simulink model "MMC_detector"  (R2022b)
settings: Solver=VariableStepAuto  StartTime=0.0  StopTime=0.6  RelTol=1e-3
undefined symbols (not defined in the file or in its folder): Atk1, Atk2, Atk3, DiscIntNeverNeededParam, plecs, Tatk1, Tatk2, Ti, Ts, Tstop
libraries: simulink x6
settings Model: Creator=Asus  LastModifiedBy=ben19
settings DebuggingCC: UnconnectedInputMsg=warning  UnconnectedOutputMsg=warning  UnconnectedLineMsg=warning
settings ModelReferenceCC: EnableRefExpFcnMdlSchedulingChecks=on
settings RTWCC: DLArmComputeVersion=19.05

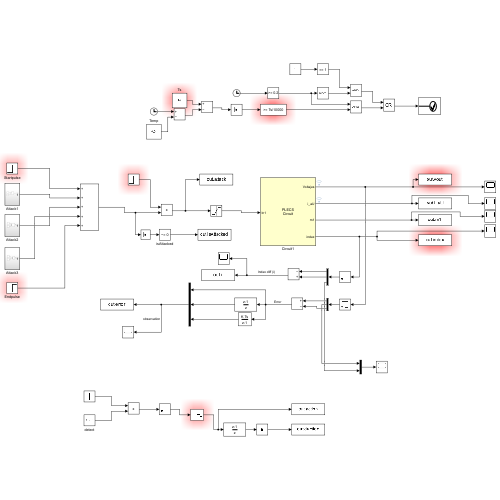
[thumbnail: Simulink's stored preview of the top-level diagram]
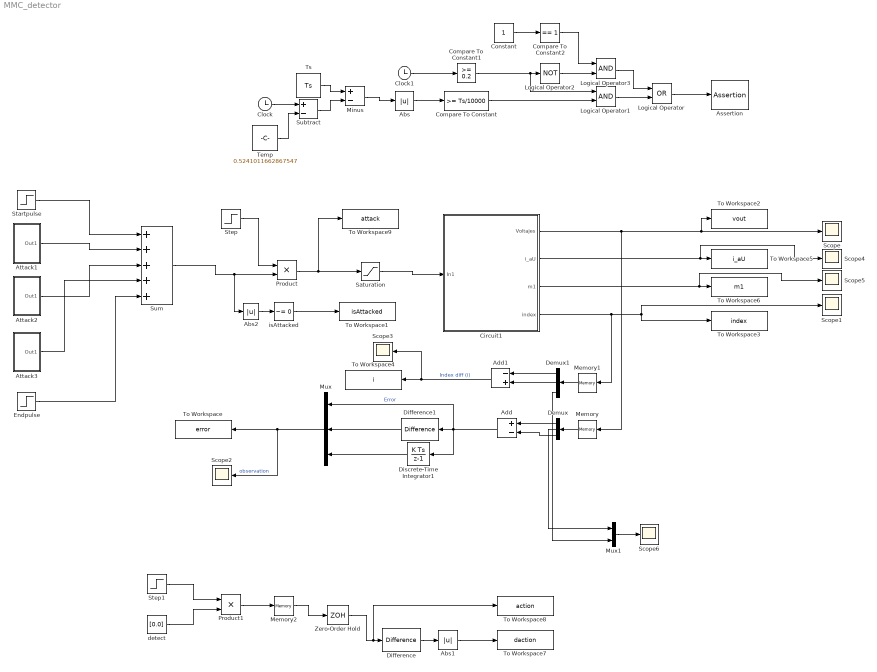
== system MMC_detector ==
  Abs : Abs  SaturateOnIntegerOverflow=off
  Abs1 : Abs  OutDataTypeStr=double  SaturateOnIntegerOverflow=off
  Abs2 : Abs  SaturateOnIntegerOverflow=off
  Add : Sum  Inputs=+-
  Add1 : Sum  Inputs=-+
  Assertion : Assertion  AssertionFailFcn=set_param(bdroot,'SimulationCommand','pause')  StopWhenAssertionFail=off
  Attack1 : Subsystem
  Attack2 : Subsystem
  Attack3 : Subsystem
  Circuit1 : Subsystem  LoadFcn=plecs('sl', 200);  InitFcn=plecs('sl', 214);  StartFcn=plecs('sl', 208);  StopFcn=plecs('sl', 209);  mask(PlecsCircuit){PLECSData=<binary blob, 67192 chars, not shown>}
      mask prompts: PLECSData "PLECS Data (Do not delete or modify!)"
      mask init:
      | % PLACE CUSTOM INITIALIZATIONS ABOVE
      | % DO NOT REMOVE
      | plecs('sl', 215);
      | % DO NOT REMOVE
      settings: CopyFcn=plecs('sl', 203);  DeleteFcn=plecs('sl', 205);  UndoDeleteFcn=plecs('sl', 206);  PreSaveFcn=plecs('sl', 211);  PostSaveFcn=plecs('sl', 201);  NameChangeFcn=plecs('sl', 210);  DestroyFcn=plecs('sl', 207);  PreCopyFcn=plecs('sl', 216);  OpenFcn=plecs('sl', 202);  ErrorFcn=plerrorfcn
      mask Help: web(['file:///' fullfile(plecsdoc, 'creatingacircuit.html')])
      mask Display: disp('PLECS\nCircuit')
  Clock : Clock
  Clock1 : Clock
  Compare To Constant : simulink/Logic and Bit Operations/Compare To Constant  relop=>=  const=Ts/10000  OutDataTypeStr=boolean
  Compare To Constant1 : simulink/Logic and Bit Operations/Compare To Constant  relop=>=  const=0.2  OutDataTypeStr=boolean
  Compare To Constant2 : simulink/Logic and Bit Operations/Compare To Constant  relop===  const=1  OutDataTypeStr=boolean
  Constant : Constant
  Demux : Demux  Outputs=3
  Demux1 : Demux  Outputs=3
  Difference : simulink/Discrete/Difference  ICPrevInput=0.0  OutMin=[]  OutMax=[]  OutDataType=fixdt(1, 16)  OutScaling=2^-10  DoSatur=off
  Difference1 : simulink/Discrete/Difference  ICPrevInput=0.0  OutMin=[]  OutMax=[]  OutDataType=fixdt(1, 16)  OutScaling=2^-10  DoSatur=off
  Discrete-Time Integrator1 : DiscreteIntegrator  SampleTime=-1  ICPrevOutput=DiscIntNeverNeededParam  ICPrevScaledInput=DiscIntNeverNeededParam
  Endpulse : Step  Time=Tstop  SampleTime=0
  Logical Operator : Logic  Operator=OR  AllPortsSameDT=off  OutDataTypeStr=boolean
  Logical Operator1 : Logic  AllPortsSameDT=off  OutDataTypeStr=boolean
  Logical Operator2 : Logic  Operator=NOT  AllPortsSameDT=off  OutDataTypeStr=boolean
  Logical Operator3 : Logic  AllPortsSameDT=off  OutDataTypeStr=boolean
  Memory : Memory
  Memory1 : Memory
  Memory2 : Memory
  Minus : Sum  Inputs=+-
  Mux : Mux  Inputs=3
  Mux1 : Mux  Inputs=2
  Product : Product
  Product1 : Product
  Saturation : Saturate  UpperLimit=50.0  LowerLimit=-50.0
  Scope{,1..6} (7 alike) : Scope
  Startpulse : Step  Time=Ti  SampleTime=0
  Step : Step  Time=Ti  SampleTime=0
  Step1 : Step  Time=0.2  SampleTime=0
  Subtract : Sum  Inputs=+-
  Sum : Sum  Inputs=+++++
  Temp : Constant  Value=0.5241011662867547
  To Workspace : ToWorkspace  VariableName=error  SampleTime=-1
      settings: Save2DSignal=2-D array (concatenate along first dimension)
  To Workspace1 : ToWorkspace  VariableName=isAttacked  SampleTime=-1
  To Workspace2 : ToWorkspace  VariableName=vout  SaveFormat=Timeseries  SampleTime=Ts
      settings: Save2DSignal=2-D array (concatenate along first dimension)
  To Workspace3 : ToWorkspace  VariableName=index  SampleTime=Ts
      settings: Save2DSignal=2-D array (concatenate along first dimension)
  To Workspace4 : ToWorkspace  VariableName=i  SampleTime=-1
      settings: Save2DSignal=2-D array (concatenate along first dimension)
  To Workspace5 : ToWorkspace  VariableName=i_aU  SampleTime=-1
      settings: Save2DSignal=2-D array (concatenate along first dimension)
  To Workspace6 : ToWorkspace  VariableName=m1  SampleTime=-1
      settings: Save2DSignal=2-D array (concatenate along first dimension)
  To Workspace7 : ToWorkspace  VariableName=daction  SampleTime=-1
  To Workspace8 : ToWorkspace  VariableName=action  SampleTime=-1
  To Workspace9 : ToWorkspace  VariableName=attack  SaveFormat=Timeseries  SampleTime=-1
  Ts : Constant  Value=Ts
  Zero-Order Hold : ZeroOrderHold  SampleTime=Ts
  detect : Constant  Value=[0.0]
  isAttacked : simulink/Logic and Bit Operations/Compare To Zero  relop=~=  OutDataTypeStr=boolean
  wires:
  Circuit1/1(Voltajes) -> Scope/1, To Workspace2/1, Memory/1
  Circuit1/4(index) -> Memory1/1, To Workspace3/1, Scope1/1
  Memory/1 -> Demux/1
  Demux/1 -> Add/1
  Add/1 -> Discrete-Time Integrator1/1, Difference1/1, Mux/1  "Error"
  Discrete-Time Integrator1/1 -> Mux/3
  Demux/3 -> Add/2
  Mux/1 -> To Workspace/1, Scope2/1  "observation"
  Memory1/1 -> Demux1/1
  Demux1/2 -> Add1/2
  Demux1/1 -> Add1/1
  Add1/1 -> To Workspace4/1, Scope3/1  "Index diff (i)"
  Circuit1/2(i_aU) -> Scope4/1, To Workspace5/1
  Circuit1/3(m1) -> Scope5/1, To Workspace6/1
  Difference1/1 -> Mux/2
  Demux1/3 -> Mux1/2
  Demux/2 -> Mux1/1
  Mux1/1 -> Scope6/1
  Step1/1 -> Product1/1
  detect/1 -> Product1/2
  Product1/1 -> Memory2/1
  Difference/1 -> Abs1/1
  Logical Operator1/1 -> Logical Operator/2
  Compare To Constant/1 -> Logical Operator1/2
  Logical Operator3/1 -> Logical Operator/1
  Abs/1 -> Compare To Constant/1
  Compare To Constant2/1 -> Logical Operator3/1
  Minus/1 -> Abs/1
  Clock1/1 -> Compare To Constant1/1
  Logical Operator/1 -> Assertion/1
  Clock/1 -> Subtract/1
  Ts/1 -> Minus/1
  Compare To Constant1/1 -> Logical Operator2/1, Logical Operator1/1
  Temp/1 -> Subtract/2
  Subtract/1 -> Minus/2
  Logical Operator2/1 -> Logical Operator3/2
  Constant/1 -> Compare To Constant2/1
  Abs2/1 -> isAttacked/1
  isAttacked/1 -> To Workspace1/1
  Saturation/1 -> Circuit1/1(In1)
  Step/1 -> Product/1
  Product/1 -> To Workspace9/1, Saturation/1
  Memory2/1 -> Zero-Order Hold/1
  Zero-Order Hold/1 -> To Workspace8/1, Difference/1
  Startpulse/1 -> Sum/1
  Attack1/1(Out1) -> Sum/2
  Attack2/1(Out1) -> Sum/3
  Attack3/1(Out1) -> Sum/4
  Endpulse/1 -> Sum/5
  Sum/1 -> Abs2/1, Product/2
  Abs1/1 -> To Workspace7/1

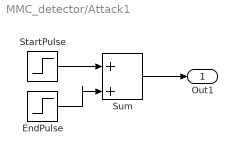
== system MMC_detector/Attack1 ==
  EndPulse : Step  Time=Ti+Tatk1  After=-Atk1  SampleTime=0
  StartPulse : Step  Time=Ti  After=Atk1  SampleTime=0
  Sum : Sum
  Out1 : Outport
  wires:
  StartPulse/1 -> Sum/1
  EndPulse/1 -> Sum/2
  Sum/1 -> Out1/1

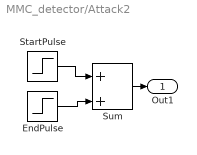
== system MMC_detector/Attack2 ==
  EndPulse : Step  Time=Ti+Tatk1+Tatk2  After=-Atk2  SampleTime=0
  StartPulse : Step  Time=Ti+Tatk1  After=Atk2  SampleTime=0
  Sum : Sum
  Out1 : Outport
  wires:
  Sum/1 -> Out1/1
  StartPulse/1 -> Sum/1
  EndPulse/1 -> Sum/2

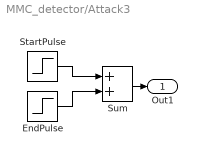
== system MMC_detector/Attack3 ==
  EndPulse : Step  Time=Tstop  After=-Atk3  SampleTime=0
  StartPulse : Step  Time=Ti+Tatk1+Tatk2  After=Atk3  SampleTime=0
  Sum : Sum
  Out1 : Outport
  wires:
  StartPulse/1 -> Sum/1
  Sum/1 -> Out1/1
  EndPulse/1 -> Sum/2

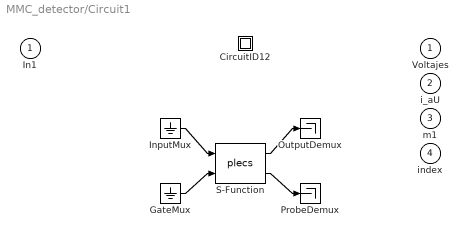
== system MMC_detector/Circuit1 ==
  In1 : Inport  PortDimensions=1
  " CircuitID12 " : Subsystem
  " GateMux " : Ground
  " InputMux " : Ground
  " OutputDemux " : Terminator
  " ProbeDemux " : Terminator
  " S-Function " : S-Function  FunctionName=plecs  SFunctionDeploymentMode=off  EnableBusSupport=off
  Voltajes : Outport  PortDimensions=3
  i_aU : Outport  Port=2  PortDimensions=1
  m1 : Outport  Port=3  PortDimensions=1
  index : Outport  Port=4  PortDimensions=3
  wires:
  " InputMux "/1 -> " S-Function "/1
  " GateMux "/1 -> " S-Function "/2
  " S-Function "/1 -> " OutputDemux "/1
  " S-Function "/2 -> " ProbeDemux "/1

== system MMC_detector/Circuit1/ CircuitID12  ==
